simulink subsystem "test"  (R2021a)
settings: Solver=VariableStepAuto  StartTime=0.0  StopTime=10.0  RelTol=1e-3
settings Model: Creator=Admin  LastModifiedBy=Admin

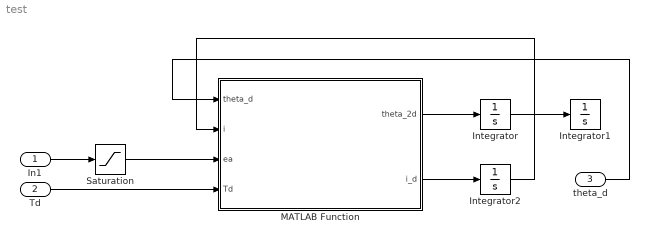
== system test ==
  In1 : Inport
  Td : Inport  Port=2
  theta_d : Inport  Port=3
  Integrator : Integrator
  Integrator1 : Integrator
  Integrator2 : Integrator
  MATLAB Function : MATLAB Function  TreatAsAtomicUnit=on
  Saturation : Saturate
  wires:
  In1/1 -> Saturation/1
  MATLAB Function/1(theta_2d) -> Integrator/1
  Integrator2/1 -> MATLAB Function/2(i)
  Td/1 -> MATLAB Function/4(Td)
  Saturation/1 -> MATLAB Function/3(ea)
  Integrator/1 -> Integrator1/1
  theta_d/1 -> MATLAB Function/1(theta_d)
  MATLAB Function/2(i_d) -> Integrator2/1

== matlab function test/MATLAB Function ==
  data: theta_d input; theta_2d output; i input; ea input; Td input; i_d output
function [theta_2d,i_d] = DC_Motor(theta_d,i,ea,Td)
%% Declare the parameters
Ra=2;
La=0.5;
Jm=0.02;
Dm=0.002953;
Kt=1.28;
Kb=0.0015;
%% System differential equations:
i_d=1/La*ea-Kb*La-theta_d-Ra/La*i;
theta_2d=Kt/Jm*i-Dm/Jm*theta_d-Td;
